simulink model "receiveDBPSK____PLUTO_SDR"  (R2022a)
settings: Solver=VariableStepAuto  StartTime=0.0  StopTime=15  RelTol=1e-3
undefined symbols (not defined in the file or in its folder): designMultirateFIR, Fs, ip, usb
libraries: plutoradiolib x1, dsparch4 x1, dspmlti4 x1, commfilt2 x1, sdrrlib x1, simulink x1, commsync2 x1
settings Model: Creator=Nithish  LastModifiedBy=Nithish

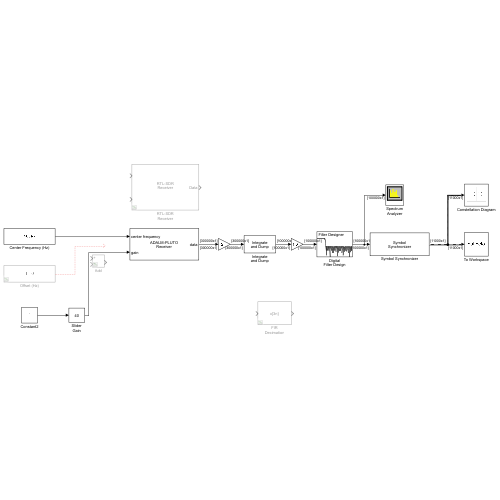
[thumbnail: Simulink's stored preview of the top-level diagram]
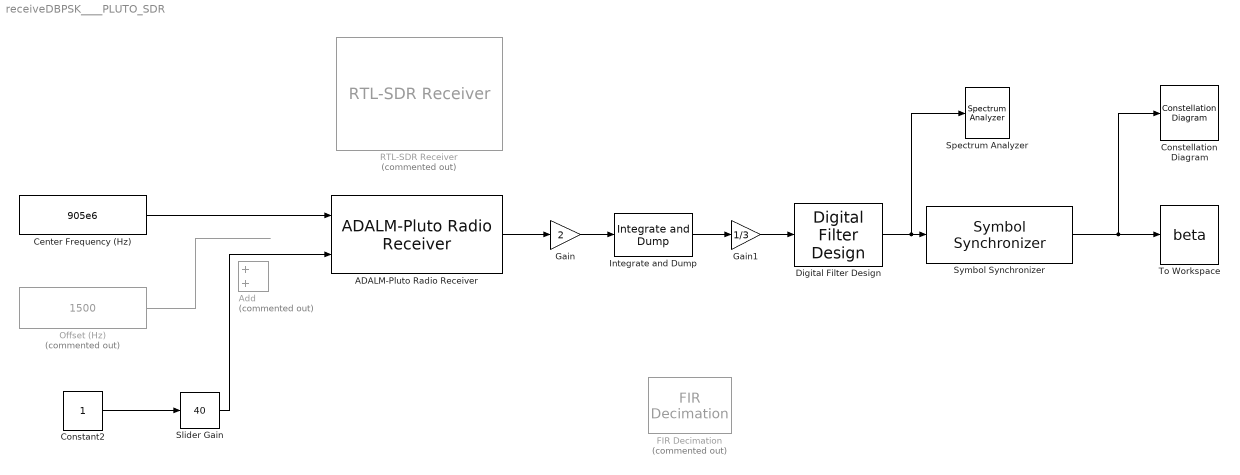
== system receiveDBPSK____PLUTO_SDR ==
  ADALM-Pluto Radio Receiver : plutoradiolib/ADALM-Pluto Radio Receiver  RadioID=usb:0  uri=ip:10.0.0.200  CenterFrequencySource=Input Port  CenterFrequency=2.4e9  GainSource=AGC Slow Attack  GainSourceBlock=Input Port  Gain=10  ChannelMapping=1  BasebandSampleRate=240e3  OutputDataType=single  SamplesPerFrame=300000  OverflowOutputPort=off  EnableBurstMode=off  NumFramesInBurst=1  ShowAdvancedProperties=off  UseCustomFilter=off  filtPathRates=[737280000 11520000 3840000 1920000 960000 240000]  filtCoefficients=[-192 82 85 -215 228 -102 -110 290 -318 145 160 -426 471 -215 -238 633 -697 318 349 -923 1009 -457 -498 1309 -1423 640 693 -1812 1959 -876 -945 2458 -2647 1180 1268 -3290 3534 -1572 -1688 4375 -4698 2091 2247 -5836 6284 -2807 -3031 7918 -8588 3870 4225 -11182 12324 -5662 -6330 17255 -19735 9507 11312 -33568 43355 -25227 -42139 305542 305542 -42139 -25227 43355 -33568 11312 9507 -19735 17255 -6330 -5662 12324 -11182 4225 3870 -8588 7918 -3031 -2807 6284 -5836 2247 2091 -4698 4375 -1688 -1572 3534 -3290 1268 1180 -2647 2458 -945 -876 1959 -1812 693 640 -1423 1309 -498 -457 1009 -923 349 318 -697 633 -238 -215 471 -426 160 145 -318 290 -110 -102 228 -215 85 82 -192]  filtCoefficientSize=128  filtDecimInterpFactor=4  filtGain=-12  filtRFBandwidth=18000000  filterConfigStruct=struct()  EnableQuadratureCorrection=on  EnableRFDCCorrection=on  EnableBasebandDCCorrection=on  FrequencyCorrection=0  OverrideSampleTime=off  SampleTime=0.02  DataTimeout=Inf  ENSMPinControlMode=None  BISTLoopbackMode=Disabled  BISTToneInject=Disabled  BISTSignalGen=PRBS  BISTToneFreq=Fs/32  BISTToneLevel=0
      settings: SourceProductBaseCode=PLUTO
  Add : Sum  Commented=on
  Center Frequency (Hz) : Constant  Value=905e6
  Constant2 : Constant
  Constellation Diagram : ConstellationDiagram  WindowPosition=[79.000000,155.000000,600.000000,600.000000,]  Visible=on  ScopeFrameLocation=window  ReferenceConstellation=BPSK  DefaultConfigurationName=comm.scopes.ConstellationDiagramBlockCfg
  Digital Filter Design : dsparch4/Digital Filter Design  mwdsp_browser_bugfix_var=off
  FIR Decimation : dspmlti4/FIR Decimation  Commented=on  FilterSource=Auto  h=designMultirateFIR(1,2)  D=3  filtStruct=Direct form  FilterObject=FDECIM  framing=Allow multirate processing  inputOffset=0  outputBufInitCond=0  roundingMode=Floor  overflowMode=off  firstCoeffDataTypeStr=Inherit: Same word length as input  firstCoeffMin=[]  firstCoeffMax=[]  firstCoeffLastDataTypeStr=Inherit: Same word length as input  outputDataTypeStr=Inherit: Same as accumulator  outputMin=[]  outputMax=[]  outputLastDataTypeStr=Inherit: Same as accumulator
  Gain : Gain  Gain=2
  Gain1 : Gain  Gain=1/3
  Integrate and Dump : commfilt2/Integrate and Dump  obssamples=3  offsetsamples=0  nodump=off  roundingMode=Floor  overflowMode=off  outputDataTypeStr=Inherit: Same as accumulator  outputLastDataTypeStr=Inherit: Same as accumulator
  Offset (Hz) : Constant  Commented=on  Value=1500
  RTL-SDR Receiver : sdrrlib/RTL-SDR Receiver  Commented=on  IPAddress=0  CenterFrequencySource=Input port  CenterFrequency=102.5e6  GainSource=Input port  Gain=0  ADCRate=240e3  FrequencyCorrection=0  LostSamplesOutputPort=off  LatencyOutputPort=off  OutputDataType=single  FrameLength=30000  EnableBurstMode=off  NumFramesInBurst=20  sobjType=sdrr.internal.SDRRTLReceiverSL  dataUDPPort=-1  ctrlUDPPort=-1  subDeviceList=nosubdev  sdrBlockType=SDRBlockTypeSLT.SDRRxBlock  requester=UNUSED_BY_SFCN  sdrExecutionMode=SDRExecutionModeSLT.ExecModeHW  BypassUserLogic=off  DecimatorSelect=DDC decimator  SourceSelect=RF data  SineAmplitude=16000  EnableInternalClock=off  BypassIQBalance=off  IFBandwidth=40e6  ADCRateSource=Dialog  IntermediateFrequency=0  DecimationFactorSource=Dialog  DecimationFactor=512  RFFrequencyIsTunable=logical(1)  SampleTime=(30000)/(240e3)  IFBandwidthSource=Dialog  SineFrequency=30000  BypassDCBlockingFilter=off  IntermediateFrequencySource=Dialog  IQBalanceCoefficients=64  SkipAllHardwareResetAndInitialization=off  EnableIQCalibrationTable=on  CacheIQCalibrationTable=off  EnableOffsetTuning=off  EnableRTLAGC=off  EnableTestMode=off  EnableTunerAGC=off  FrequencyCorrectionSource=Dialog  NumMLBuffers=128  NumUSBBuffers=16  RTLCrystalFrequency=28800000  TunerCrystalFrequency=28800000
      settings: SourceProductBaseCode=RTLSDR
  Slider Gain : simulink/Math Operations/Slider Gain  gain=40  low=0  high=500
  Spectrum Analyzer : SpectrumAnalyzer
  Symbol Synchronizer : commsync2/Symbol Synchronizer  Modulation=PAM/PSK/QAM  TimingErrorDetector=Zero-Crossing (decision-directed)  SamplesPerSymbol=10  DampingFactor=1  NormalizedLoopBandwidth=0.01  DetectorGain=2.7  TimingErrorOutputPort=off  SimulateUsing=Code generation
      settings: SourceProductBaseCode=CM
  To Workspace : ToWorkspace  VariableName=beta  SaveFormat=Structure  SampleTime=-1
      settings: Save2DSignal=2-D array (concatenate along first dimension)
  wires:
  Offset (Hz)/1 -> ?
  Constant2/1 -> Slider Gain/1
  Center Frequency (Hz)/1 -> ADALM-Pluto Radio Receiver/1
  Integrate and Dump/1 -> Gain1/1
  Digital Filter Design/1 -> Symbol Synchronizer/1, Spectrum Analyzer/1
  Symbol Synchronizer/1 -> To Workspace/1, Constellation Diagram/1
  ADALM-Pluto Radio Receiver/1 -> Gain/1
  Gain/1 -> Integrate and Dump/1
  Slider Gain/1 -> ADALM-Pluto Radio Receiver/2
  Gain1/1 -> Digital Filter Design/1
